simulink model "ForwardKinematics"  (R2023a)
settings: Solver=VariableStepAuto  StartTime=0.0  StopTime=5  RelTol=1e-3
values from neighbouring files (symbols this model uses):
  m = [4.043687892216430,4.088351020081470,2.975514330882000,2.005251413706830,1.580964077451070,0.312204788418883]    [Alternative_Approach_for_Jacobian.m]    (also in Dynamics6DOF_code.m)
undefined symbols (not defined in the file or in its folder): sigbuilder_block, X, Y, Z
libraries: sm_lib x61, nesl_utility x13, simulink_extras x6, robotmaniplib x3, robotcorelib x2
(part 2 of 2)

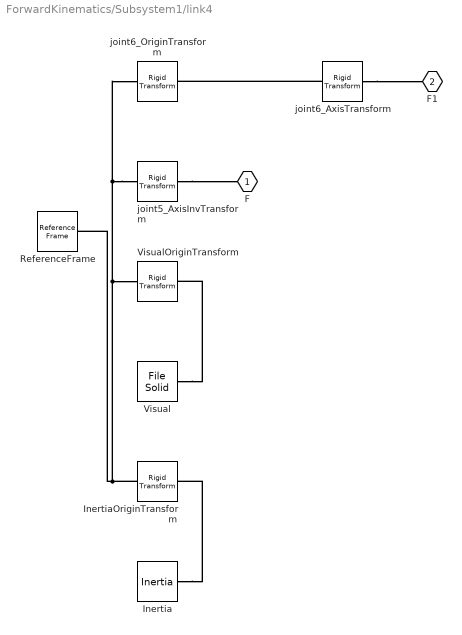
== system ForwardKinematics/Subsystem1/link4 ==
  Inertia : sm_lib/Body Elements/Inertia  InertiaType=Custom  Mass=1.93952788406336  MassUnits=kg  CenterOfMass=[0, 0, 0]  CenterOfMassUnits=m  MomentsOfInertia=[0.00155390886602976, 0.00197625240925502, 0.00139914012504898]  MomentsOfInertiaUnits=kg*m^2  ProductsOfInertia=[-0.000238629251977827, 2.66730188215764e-06, -2.69206560401887e-06]  ProductsOfInertiaUnits=kg*m^2  GraphicType=None  MarkerShape=Inertia  MarkerSize=20  GraphicVisPropType=SimpleVisualProperties  GraphicDiffuseColor=[0.5 0.5 0.5]  GraphicSpecularColor=[0.5 0.5 0.5 1.0]  GraphicAmbientColor=[0.15 0.15 0.15 1.0]  GraphicEmissiveColor=[0.0 0.0 0.0 1.0]  GraphicShininess=75  GraphicOpacity=1.0
  InertiaOriginTransform : sm_lib/Frames and Transforms/Rigid Transform  TranslationMethod=Cartesian  TranslationStandardOffset=0  TranslationStandardOffsetUnits=m  TranslationStandardAxis=+Z  TranslationCartesianOffset=[0.00193589454404341, 0.0412277276852661, -0.00711984165498196]  TranslationCartesianOffsetUnits=m  TranslationROffset=0  TranslationROffsetUnits=m  TranslationZOffset=0  TranslationZOffsetUnits=m  TranslationThetaOffset=0  TranslationThetaOffsetUnits=deg  RotationMethod=RotationSequence  RotationAngleUnits=deg  RotationStandardAxis=+Z  RotationAngle=0.0  RotationArbitraryAxis=[0 0 1]  FollAlignAxisA=+X  BaseAlignAxisA=+Y  FollAlignAxisB=+Y  BaseAlignAxisB=+Z  RotationSequenceAxes=BaseAxes  RotationSequence=XYZ  RotationSequenceAngles=[0, 0, 0]  RotationSequenceAnglesUnits=rad  RotationMatrix=[1 0 0; 0 1 0; 0 0 1]  Quaternion=[1 0 0 0]
  ReferenceFrame : sm_lib/Frames and Transforms/Reference Frame
  Visual : sm_lib/Body Elements/File Solid  ExtGeomFileName=PickandPlace_Assembly/meshes/link4.STL  UnitType=Custom  ExtGeomFileUnits=m  StepReaderType=HEX  ExportConvexHullGeometry=off  InertiaType=Custom  Mass=0  MassUnits=kg  CenterOfMass=[0, 0, 0]  CenterOfMassUnits=m  MomentsOfInertia=[0, 0, 0]  MomentsOfInertiaUnits=kg*m^2  ProductsOfInertia=[0, 0, 0]  ProductsOfInertiaUnits=kg*m^2  BasedOnType=DensityFromFile  Density=1000  DensityUnits=kg/m^3  DoExposeReferenceFrame=on  SerializedFrames=<Frames/>  GraphicType=FromGeometry  MarkerShape=Sphere  MarkerSize=10  GraphicVisPropType=SimpleVisualProperties  GraphicDiffuseColor=[0.752941176470588, 0.752941176470588, 0.752941176470588]  GraphicSpecularColor=[0.5 0.5 0.5 1.0]  GraphicAmbientColor=[0.15 0.15 0.15 1.0]  GraphicEmissiveColor=[0.0 0.0 0.0 1.0]  GraphicShininess=75  GraphicOpacity=1
  VisualOriginTransform : sm_lib/Frames and Transforms/Rigid Transform  TranslationMethod=Cartesian  TranslationStandardOffset=0  TranslationStandardOffsetUnits=m  TranslationStandardAxis=+Z  TranslationCartesianOffset=[0, 0, 0.132]  TranslationCartesianOffsetUnits=m  TranslationROffset=0  TranslationROffsetUnits=m  TranslationZOffset=0  TranslationZOffsetUnits=m  TranslationThetaOffset=0  TranslationThetaOffsetUnits=deg  RotationMethod=RotationSequence  RotationAngleUnits=deg  RotationStandardAxis=+Z  RotationAngle=0.0  RotationArbitraryAxis=[0 0 1]  FollAlignAxisA=+X  BaseAlignAxisA=+Y  FollAlignAxisB=+Y  BaseAlignAxisB=+Z  RotationSequenceAxes=BaseAxes  RotationSequence=XYZ  RotationSequenceAngles=[0, 0, 0]  RotationSequenceAnglesUnits=rad  RotationMatrix=[1 0 0; 0 1 0; 0 0 1]  Quaternion=[1 0 0 0]
  joint5_AxisInvTransform : sm_lib/Frames and Transforms/Rigid Transform  TranslationMethod=Cartesian  TranslationStandardOffset=0  TranslationStandardOffsetUnits=m  TranslationStandardAxis=+Z  TranslationCartesianOffset=[0, 0, 0]  TranslationCartesianOffsetUnits=m  TranslationROffset=0  TranslationROffsetUnits=m  TranslationZOffset=0  TranslationZOffsetUnits=m  TranslationThetaOffset=0  TranslationThetaOffsetUnits=deg  RotationMethod=ArbitraryAxis  RotationAngleUnits=rad  RotationStandardAxis=+Z  RotationAngle=0  RotationArbitraryAxis=[1, 0, 0]  FollAlignAxisA=+X  BaseAlignAxisA=+Y  FollAlignAxisB=+Y  BaseAlignAxisB=+Z  RotationSequenceAxes=FollowerAxes  RotationSequence=XYX  RotationSequenceAngles=[0 0 0]  RotationSequenceAnglesUnits=deg  RotationMatrix=[1 0 0; 0 1 0; 0 0 1]  Quaternion=[1 0 0 0]
  joint6_AxisTransform : sm_lib/Frames and Transforms/Rigid Transform  TranslationMethod=Cartesian  TranslationStandardOffset=0  TranslationStandardOffsetUnits=m  TranslationStandardAxis=+Z  TranslationCartesianOffset=[0, 0, 0]  TranslationCartesianOffsetUnits=m  TranslationROffset=0  TranslationROffsetUnits=m  TranslationZOffset=0  TranslationZOffsetUnits=m  TranslationThetaOffset=0  TranslationThetaOffsetUnits=deg  RotationMethod=ArbitraryAxis  RotationAngleUnits=rad  RotationStandardAxis=+Z  RotationAngle=0  RotationArbitraryAxis=[1, 0, 0]  FollAlignAxisA=+X  BaseAlignAxisA=+Y  FollAlignAxisB=+Y  BaseAlignAxisB=+Z  RotationSequenceAxes=FollowerAxes  RotationSequence=XYX  RotationSequenceAngles=[0 0 0]  RotationSequenceAnglesUnits=deg  RotationMatrix=[1 0 0; 0 1 0; 0 0 1]  Quaternion=[1 0 0 0]
  joint6_OriginTransform : sm_lib/Frames and Transforms/Rigid Transform  TranslationMethod=Cartesian  TranslationStandardOffset=0  TranslationStandardOffsetUnits=m  TranslationStandardAxis=+Z  TranslationCartesianOffset=[0, 0, 0.132]  TranslationCartesianOffsetUnits=m  TranslationROffset=0  TranslationROffsetUnits=m  TranslationZOffset=0  TranslationZOffsetUnits=m  TranslationThetaOffset=0  TranslationThetaOffsetUnits=deg  RotationMethod=RotationSequence  RotationAngleUnits=deg  RotationStandardAxis=+Z  RotationAngle=0.0  RotationArbitraryAxis=[0 0 1]  FollAlignAxisA=+X  BaseAlignAxisA=+Y  FollAlignAxisB=+Y  BaseAlignAxisB=+Z  RotationSequenceAxes=BaseAxes  RotationSequence=XYZ  RotationSequenceAngles=[-1.5707963267949, 0, 0]  RotationSequenceAnglesUnits=rad  RotationMatrix=[1 0 0; 0 1 0; 0 0 1]  Quaternion=[1 0 0 0]
  F : PMIOPort  Side=Left
  F1 : PMIOPort  Port=2  Side=Right
  connections:
  Inertia/RConn1 -- InertiaOriginTransform/RConn1
  joint5_AxisInvTransform/LConn1 -- joint6_OriginTransform/LConn1 -- InertiaOriginTransform/LConn1 -- ReferenceFrame/RConn1 -- VisualOriginTransform/LConn1
  Visual/RConn1 -- VisualOriginTransform/RConn1
  joint5_AxisInvTransform/RConn1 -- F/RConn1
  joint6_AxisTransform/RConn1 -- F1/RConn1
  joint6_AxisTransform/LConn1 -- joint6_OriginTransform/RConn1

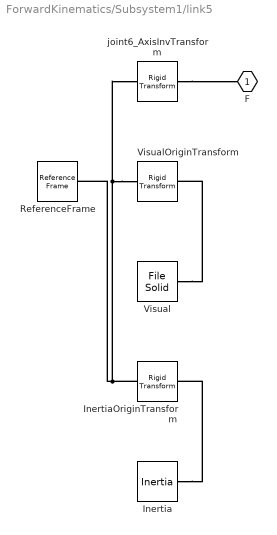
== system ForwardKinematics/Subsystem1/link5 ==
  Inertia : sm_lib/Body Elements/Inertia  InertiaType=Custom  Mass=0.312204788121022  MassUnits=kg  CenterOfMass=[0, 0, 0]  CenterOfMassUnits=m  MomentsOfInertia=[0.000111486628802788, 0.00017220756532504, 0.000149930296123144]  MomentsOfInertiaUnits=kg*m^2  ProductsOfInertia=[-2.62510399493773e-06, -6.16294543592803e-07, 1.09193037299933e-05]  ProductsOfInertiaUnits=kg*m^2  GraphicType=None  MarkerShape=Inertia  MarkerSize=20  GraphicVisPropType=SimpleVisualProperties  GraphicDiffuseColor=[0.5 0.5 0.5]  GraphicSpecularColor=[0.5 0.5 0.5 1.0]  GraphicAmbientColor=[0.15 0.15 0.15 1.0]  GraphicEmissiveColor=[0.0 0.0 0.0 1.0]  GraphicShininess=75  GraphicOpacity=1.0
  InertiaOriginTransform : sm_lib/Frames and Transforms/Rigid Transform  TranslationMethod=Cartesian  TranslationStandardOffset=0  TranslationStandardOffsetUnits=m  TranslationStandardAxis=+Z  TranslationCartesianOffset=[0.000634869948304639, 0.00391637711045545, 0.0604907685184927]  TranslationCartesianOffsetUnits=m  TranslationROffset=0  TranslationROffsetUnits=m  TranslationZOffset=0  TranslationZOffsetUnits=m  TranslationThetaOffset=0  TranslationThetaOffsetUnits=deg  RotationMethod=RotationSequence  RotationAngleUnits=deg  RotationStandardAxis=+Z  RotationAngle=0.0  RotationArbitraryAxis=[0 0 1]  FollAlignAxisA=+X  BaseAlignAxisA=+Y  FollAlignAxisB=+Y  BaseAlignAxisB=+Z  RotationSequenceAxes=BaseAxes  RotationSequence=XYZ  RotationSequenceAngles=[0, 0, 0]  RotationSequenceAnglesUnits=rad  RotationMatrix=[1 0 0; 0 1 0; 0 0 1]  Quaternion=[1 0 0 0]
  ReferenceFrame : sm_lib/Frames and Transforms/Reference Frame
  Visual : sm_lib/Body Elements/File Solid  ExtGeomFileName=PickandPlace_Assembly/meshes/link5.STL  UnitType=Custom  ExtGeomFileUnits=m  StepReaderType=HEX  ExportConvexHullGeometry=off  InertiaType=Custom  Mass=0  MassUnits=kg  CenterOfMass=[0, 0, 0]  CenterOfMassUnits=m  MomentsOfInertia=[0, 0, 0]  MomentsOfInertiaUnits=kg*m^2  ProductsOfInertia=[0, 0, 0]  ProductsOfInertiaUnits=kg*m^2  BasedOnType=DensityFromFile  Density=1000  DensityUnits=kg/m^3  DoExposeReferenceFrame=on  SerializedFrames=<Frames/>  GraphicType=FromGeometry  MarkerShape=Sphere  MarkerSize=10  GraphicVisPropType=SimpleVisualProperties  GraphicDiffuseColor=[0.752941176470588, 0.752941176470588, 0.752941176470588]  GraphicSpecularColor=[0.5 0.5 0.5 1.0]  GraphicAmbientColor=[0.15 0.15 0.15 1.0]  GraphicEmissiveColor=[0.0 0.0 0.0 1.0]  GraphicShininess=75  GraphicOpacity=1
  VisualOriginTransform : sm_lib/Frames and Transforms/Rigid Transform  TranslationMethod=Cartesian  TranslationStandardOffset=0  TranslationStandardOffsetUnits=m  TranslationStandardAxis=+Z  TranslationCartesianOffset=[0, 0, 0.050999]  TranslationCartesianOffsetUnits=m  TranslationROffset=0  TranslationROffsetUnits=m  TranslationZOffset=0  TranslationZOffsetUnits=m  TranslationThetaOffset=0  TranslationThetaOffsetUnits=deg  RotationMethod=RotationSequence  RotationAngleUnits=deg  RotationStandardAxis=+Z  RotationAngle=0.0  RotationArbitraryAxis=[0 0 1]  FollAlignAxisA=+X  BaseAlignAxisA=+Y  FollAlignAxisB=+Y  BaseAlignAxisB=+Z  RotationSequenceAxes=BaseAxes  RotationSequence=XYZ  RotationSequenceAngles=[0, 0, 0]  RotationSequenceAnglesUnits=rad  RotationMatrix=[1 0 0; 0 1 0; 0 0 1]  Quaternion=[1 0 0 0]
  joint6_AxisInvTransform : sm_lib/Frames and Transforms/Rigid Transform  TranslationMethod=Cartesian  TranslationStandardOffset=0  TranslationStandardOffsetUnits=m  TranslationStandardAxis=+Z  TranslationCartesianOffset=[0, 0, 0]  TranslationCartesianOffsetUnits=m  TranslationROffset=0  TranslationROffsetUnits=m  TranslationZOffset=0  TranslationZOffsetUnits=m  TranslationThetaOffset=0  TranslationThetaOffsetUnits=deg  RotationMethod=ArbitraryAxis  RotationAngleUnits=rad  RotationStandardAxis=+Z  RotationAngle=0  RotationArbitraryAxis=[1, 0, 0]  FollAlignAxisA=+X  BaseAlignAxisA=+Y  FollAlignAxisB=+Y  BaseAlignAxisB=+Z  RotationSequenceAxes=FollowerAxes  RotationSequence=XYX  RotationSequenceAngles=[0 0 0]  RotationSequenceAnglesUnits=deg  RotationMatrix=[1 0 0; 0 1 0; 0 0 1]  Quaternion=[1 0 0 0]
  F : PMIOPort  Side=Left
  connections:
  Inertia/RConn1 -- InertiaOriginTransform/RConn1
  VisualOriginTransform/LConn1 -- joint6_AxisInvTransform/LConn1 -- InertiaOriginTransform/LConn1 -- ReferenceFrame/RConn1
  Visual/RConn1 -- VisualOriginTransform/RConn1
  joint6_AxisInvTransform/RConn1 -- F/RConn1

== matlab function ForwardKinematics/MATLAB Function1 ==
  data: th1 input; J output; th2 input; th3 input; th4 input; th5 input; th6 input
function J = jacobian6DOF(th1, th2, th3, th4, th5, th6)
    % Define the link parameters
    d1 = 0.179; a2 = 0.410; a3 = 0.340; d4 = 0.188; d5 = 0.132; d6 = 0.0;
    
    % Define the trigonometric functions
    c1 = cos(th1); c2 = cos(th2); c3 = cos(th3); c4 = cos(th4); c5 = cos(th5); c6 = cos(th6);
    s1 = sin(th1); s2 = sin(th2); s3 = sin(th3); s4 = sin(th4); s5 = sin(th5); s6 = sin(th6);
    
    % Compute rotation matrices for each joint
    c234 = cos(th2 + th3 + th4);
    s234 = sin(th2 + th3 + th4);
    c23 = cos(th2 + th3);
    s23 = sin(th2 + th3);
    
    % Position and rotation components
    r11 = (c1*c234*c5*c6 ) + (c6*s1*s5)- (c1*s234*s6);
    r21 = (c234*c5*c6*s1)-(c1*c6*s5)- (s1*s234*s6);
    r31 = (c5*c6*s234) + (c234*s6);
    r12 = (-c1*c234*c5*s6)-(s1*s5*s6)-(c1*c6*s234);
    r22 = (-c234*c5*s1*s6) + (c1*s5*s6 )- (c6*s1*s234);
    r32 = (-c5*s234*s6) + (c234*c6);
    r13 = (-c1*c234*s5) + (c5*s1);
    r23 = (-c234*s1*s5)- (c1*c5);
    r33 = -s234*s5;
    
    % End-effector position
    px = r13*d6 + c1*(s234*d5 + c23*a3 + c2*a2) + s1*d4 ;
    py = r23*d6 + s1*(s234*d5 + c23*a3 + c2*a2) - c1*d4 ;
    pz = r33*d6 - c234*d5 + s23*a3 + s2*a2 + d1;
    
    % Full transformation matrix
    T2 = [r11 r12 r13 px; r21 r22 r23 py; r31 r32 r33 pz; 0 0 0 1];
    
    % Jacobian matrix components (JL1 to JL6)
    JL1 = [-py; px; 0];
    JL2 = [-c1*(pz - d1); -s1*(pz - d1); s1*py + c1*px];
    JL3 = [c1*(cos(th2+th3+th4)*s5*d6 + cos(th2+th3+th4)*d5 - sin(th2+th3)*a3);
           s1*(cos(th2+th3+th4)*s5*d6 + cos(th2+th3+th4)*d5 - sin(th2+th3)*a3);
           -cos(th2+th3+th4)*s5*d6 + cos(th2+th3+th4)*d5 + cos(th2+th3)*a3];
    JL4 = [cos(th1)*(cos(th2+th3+th4)*s5*d6 + cos(th2+th3+th4)*d5);
           sin(th1)*(cos(th2+th3+th4)*s5*d6 + cos(th2+th3+th4)*d5);
           -cos(th2+th3+th4)*s5*d6 + cos(th2+th3+th4)*d5];
    JL5 = [-d6*(sin(th1)*s5 + cos(th1)*cos(th2+th3+th4)*cos(th5));
           d6*(cos(th1)*s5 - cos(th2+th3+th4)*cos(th5)*sin(th1));
           -sin(th5)*cos(th2+th3+th4)*d6];
    JL6 = [0; 0; 0];  % Typically, this term would depend on the type of manipulator
    
    % Jacobian matrix
    JL = [JL1, JL2, JL3, JL4, JL5, JL6];
    
    % Angular velocity part of the Jacobian (JA)
    JA = [0, s1, s1, s1, c1*c234, r13;
          0, -c1, -c1, -c1, s1*s234, r23;
          1, 0, 0, 0, -c234, r33];
    
    % Full Jacobian matrix (linear + angular velocity parts)
    J = [JL; JA];
    
    % Display the Jacobian matrix
    disp('Jacobian Matrix:');
    disp(J);
end

== matlab function ForwardKinematics/MATLAB Function ==
  data: T2 output; th1 input; th2 input; th3 input; th4 input; th5 input; th6 input
% % function T2  = forward6DOF(th1,th2,th3,th4,th5,th6)
% %     d1=0.179;a2=0.410;a3=0.340;d4=0.104;d5=0.089;d6=0.050;
% %     c1=cos(th1); c2=cos(th2); c5=cos(th5); c6=cos(th6);c3=cos(th3);
% %     s1=sin(th1); s2=sin(th2); s3=sin(th3);s5=sin(th5); s6=sin(th6);
% %     c234=cos(th2+th3+th4); s234=sin(th2+th3+th4); c23=cos(th2+th3); s23=sin(th2+th3);
% %     r11= c6*(s1*s5+((c1*c234- s1*s234)*c5)/2.0+((c1*c234 + s1*s234)*c5)/2.0)-(s6*((s1*c234 + c1*s234)-(s1*c234-c1*s234)))/2.0;
% %     r21= c6*(((s1*c234 + c1*s234)*c5)/2.0-c1*s5 + ((s1*c234-c1*s234)*c5)/2.0)+s6*((c1*c234-s1*s234)/2.0-(c1*c234+s1*s234)/2.0);
% %     r31= (s234*c6+ c234*s6)/2.0+s234*c5*c6-(s234*c6-c234*s6)/2.0;
% %     r12= -(c6*((s1*c234 + c1*s234)-(s1*c234- c1*s234)))/2.0-s6*(s1*s5+((c1*c234-s1*s234)*c5)/2.0+((c1*c234+s1*s234)*c5)/2.0);
% %     r22= c6*((c1*c234-s1*s234)/2.0-(c1*c234+s1*s234)/2.0)-s6*(((s1*c234+c1*s234)*c5)/2.0-c1*s5+((s1*c234-c1*s234)*c5)/2.0);
% %     r32=  (c234*c6 + s234*s6)/2.0 + (c234*c6-s234*s6)/2.0-s234*c5*s6;
% %     r13= c5*s1-((c1*c234-s1*s234)*s5)/2.0-((c1*c234 + s1*s234)*s5)/2.0;
% %     r23= -c1*c5-((s1*c234 + c1*s234)*s5)/2.0 + ((c1*s234-s1*c234)*s5)/2.0;
% %     r33=  (c234*c5-s234*s5)/2.0 -(c234*c5 + s234*s5)/2.0;
% %     px= -(d5*(s1*c234-c1*s234))/2.0+(d5*(s1*c234+c1*s234))/2.0+d4*s1-(d6*(c1*c234-s1*s234)*s5)/2.0-(d6*(c1*c234+s1*s234)*s5)/2.0 + a2*c1*c2 + d6*c5*s1 + a3*c1*c2*c3-a3*c1*s2*s3;
% %     py= -(d5*(c1*c234-s1*s234))/2.0+(d5*(c1*c234+s1*s234))/2.0-d4*c1-(d6*(s1*c234+c1*s234)*s5)/2.0-(d6*(s1*c234-c1*s234)*s5)/2.0-d6*c1*c5 + a2*c2*s1 + a3*c2*c3*s1-a3*s1*s2*s3;
% %     pz= d1 + (d6*(c234*c5-s234*s5))/2.0 + a3*(s2*c3 + c2*s3) + a2*s2- (d6*(c234*c5 + s234*s5))/2.0-d5*c234;
% % % 
% % %     T2=[r11 r12 r13 px; r21 r22 r23 py; r31 r32 r33 pz; 0 0 0 1];    
% % % end
% % 
% 
function T2  = forward6DOF(th1,th2,th3,th4,th5,th6)
    
    d1=0.179;a2=0.410;a3=0.340;d4=0.188;d5=0.132;d6=0.0;
   
    c1=cos(th1); c2=cos(th2); c5=cos(th5); c6=cos(th6);
    s1=sin(th1); s2=sin(th2); s5=sin(th5); s6=sin(th6);
    c234=cos(th2+th3+th4); s234=sin(th2+th3+th4); c23=cos(th2+th3); s23=sin(th2+th3);
    r11= (c1*c234*c5*c6 )+ (c6*s1*s5)- (c1*s234*s6);
    r21= (c234*c5*c6*s1)-(c1*c6*s5)- (s1*s234*s6);
    r31 = (c5*c6*s234) + (c234*s6);
    r12 = (-c1*c234*c5*s6)-(s1*s5*s6)-(c1*c6*s234) ;
    r22 = (-c234*c5*s1*s6) + (c1*s5*s6 )- (c6*s1*s234);
    r32 = (-c5*s234*s6) + (c234*c6);
    r13 = (-c1*c234*s5) + (c5*s1);
    r23 = (-c234*s1*s5)- (c1*c5);
    r33 = -s234*s5;
    px = r13*d6 + c1*(s234*d5 + c23*a3 + c2*a2) + s1*d4 ;
    py = r23*d6 + s1*(s234*d5 + c23*a3 + c2*a2) - c1*d4 ;
    pz = r33*d6 - c234*d5 + s23*a3 + s2*a2 + d1;

    T2=[r11 r12 r13 px; r21 r22 r23 py; r31 r32 r33 pz; 0 0 0 1];
        % Jacobian matrix JL1 to JL6 (from your given expressions)
    
end









% 
% function T2  = forward6DOF(th1,th2,th3,th4,th5,th6)
%     
%     d1=0.179;a2=0.410;a3=0.34325;d4=0.188;d5=0.12875;d6=0.050;
%     c1=cosd(th1); c2=cosd(th2); c5=cosd(th5); c6=cosd(th6);
%     s1=sind(th1); s2=sind(th2); s5=sind(th5); s6=sind(th6);
%     c234=cosd(th2+th3+th4); s234=sind(th2+th3+th4); c23=cosd(th2+th3); s23=sind(th2+th3);
%     r11= (c1*c234*c5*c6 )+ (c6*s1*s5)- (c1*s234*s6);
%     r21= (c234*c5*c6*s1)-(c1*c6*s5)- (s1*s234*s6);
%     r31 = (c5*c6*s234) + (c234*s6);
%     r12 = (-c1*c234*c5*s6)-(s1*s5*s6)-(c1*c6*s234) ;
%     r22 = (-c234*c5*s1*s6) + (c1*s5*s6 )- (c6*s1*s234);
%     r32 = (-c5*s234*s6) + (c234*c6);
%     r13 = (-c1*c234*s5) + (c5*s1);
%     r23 = (-c234*s1*s5)- (c1*c5);
%     r33 = -s234*s5;
%     px = r13*d6 + c1*(s234*d5 + c23*a3 + c2*a2) + s1*d4 ;
%     py = r23*d6 + s1*(s234*d5 + c23*a3 + c2*a2) - c1*d4 ;
%     pz = r33*d6 - c234*d5 + s23*a3 + s2*a2 + d1;
% 
%     T2=[r11 r12 r13 px; r21 r22 r23 py; r31 r32 r33 pz; 0 0 0 1]
% end
